simulink library "lib_fault_definiteness"  (R2023a)
settings: Solver=VariableStepAuto  StartTime=0.0  StopTime=10.0  RelTol=1e-3
settings Model: Creator=YXQ1WX  LastModifiedBy=xiaoqiang.yuan
settings OptimizationCC: ReuseModelBlockBuffer=off

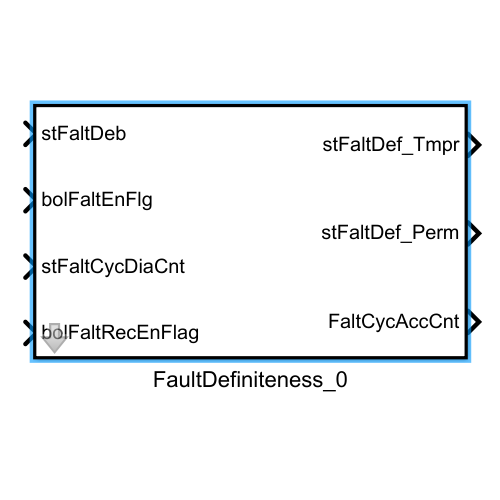
[thumbnail: Simulink's stored preview of the top-level diagram]
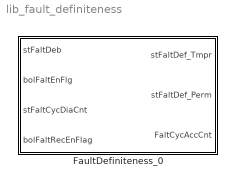
== system lib_fault_definiteness ==
  FaultDefiniteness_0 : Subsystem  TreatAsAtomicUnit=on  mask{lb_FaltWaitRecvCnt=0}
      mask prompts: lb_FaltWaitRecvCnt "FailWaitRecvryCounter"
      mask DialogControl DescGroupVar Prompt: WF control library
      mask DialogControl DescTextVar Prompt: For fault definiteness

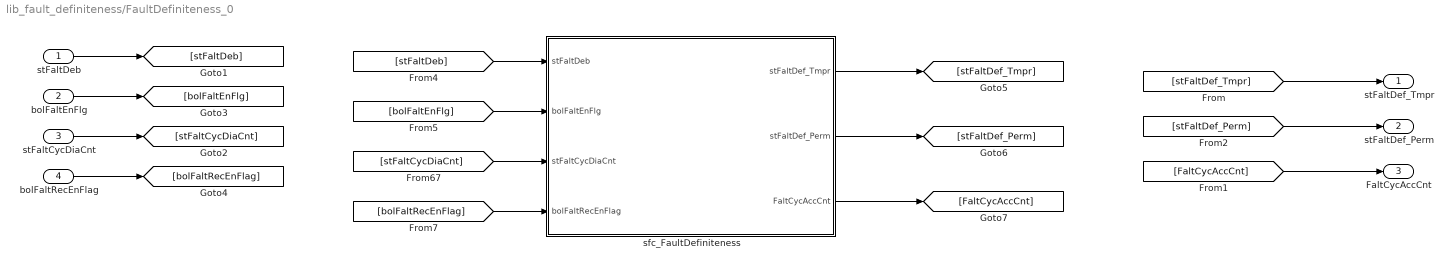
== system lib_fault_definiteness/FaultDefiniteness_0 ==
  stFaltDeb : Inport
  bolFaltEnFlg : Inport  Port=2
  stFaltCycDiaCnt : Inport  Port=3
  bolFaltRecEnFlag : Inport  Port=4
  sfc_FaultDefiniteness : Stateflow chart  TreatAsAtomicUnit=on
  stFaltDef_Tmpr : Outport
  stFaltDef_Perm : Outport  Port=2
  FaltCycAccCnt : Outport  Port=3
  wires:
  sfc_FaultDefiniteness/1(stFaltDef_Tmpr) -> [stFaltDef_Tmpr]
  sfc_FaultDefiniteness/2(stFaltDef_Perm) -> [stFaltDef_Perm]
  sfc_FaultDefiniteness/3(FaltCycAccCnt) -> [FaltCycAccCnt]
  [stFaltDeb] -> sfc_FaultDefiniteness/1(stFaltDeb)
  [bolFaltEnFlg] -> sfc_FaultDefiniteness/2(bolFaltEnFlg)
  [stFaltCycDiaCnt] -> sfc_FaultDefiniteness/3(stFaltCycDiaCnt)
  [bolFaltRecEnFlag] -> sfc_FaultDefiniteness/4(bolFaltRecEnFlag)
  stFaltDeb/1 -> [stFaltDeb]
  bolFaltEnFlg/1 -> [bolFaltEnFlg]
  stFaltCycDiaCnt/1 -> [stFaltCycDiaCnt]
  bolFaltRecEnFlag/1 -> [bolFaltRecEnFlag]
  [stFaltDef_Tmpr] -> stFaltDef_Tmpr/1
  [FaltCycAccCnt] -> FaltCycAccCnt/1
  [stFaltDef_Perm] -> stFaltDef_Perm/1

== stateflow chart lib_fault_definiteness/FaultDefiniteness_0/sfc_FaultDefiniteness ==
  state EnableDiagnosis
    state Normal
      /*Clear Bit0 Bit1*/
      en:  stFaltDef_Tmpr = false;
      stFaltDef_Perm = false;
      FaltCycAccCnt = uint8(0);
    state Confirming
      /*Set Bit0 Bit1*/
      en:  stFaltDef_Tmpr = true;
      stFaltDef_Perm = true;
      FaltCycAccCnt = FaltCycAccCnt + uint8(1);
    state Wait
      /*Set Bit0 Clear Bit1*/
      en:  stFaltDef_Tmpr = true;
      stFaltDef_Perm = false;
      FaltWaitRecvCnt = uint16(0);
      du:
      FaltWaitRecvCnt = FaltWaitRecvCnt + uint16(1);
      ex: FaltWaitRecvCnt = uint16(0);
    state Confirmed
      /*Set Bit1 Clear Bit0*/
      en:  stFaltDef_Tmpr = false;
      stFaltDef_Perm = true;
      FaltCycAccCnt = uint8(0);
    (default) -> Normal
    Normal -> (junction 181) : /*There is Fault*/
        | [stFaltDeb]
    (junction 181) -> (junction 184) [order 1] : /*Direct Confirm*/
        | [stFaltCycDiaCnt == uint8(0)]
    (junction 181) -> Confirming [order 2]
    (junction 184) -> Confirmed
    (junction 233) -> Normal
    Wait -> (junction 233) [order 2] : /*Confirm to Recovery*/
        | [FaltWaitRecvCnt > uint16(uint16(2*lb_FaltWaitRecvCnt) + uint16(100)) &&...
        | !stFaltDeb && bolFaltEnFlg]
    (junction 229) -> Normal
    Confirming -> Wait : /*There is no Fault*/
        | [!stFaltDeb]
    Wait -> (junction 212) [order 1] : /*There is Fault*/
        | [stFaltDeb]
    (junction 212) -> Confirming [order 2] : /*Need Confirm*/
    (junction 212) -> (junction 231) [order 1] : /*Fault is Confirmed*/
        | [FaltCycAccCnt >= stFaltCycDiaCnt]
    (junction 231) -> Confirmed
    Confirmed -> (junction 229) : /*Need Recovery*/
        | [bolFaltRecEnFlag &&...
        | !stFaltDeb]
  state DisableDiagnosis
    /*Clear Bit0 Bit1*/
    en:  stFaltDef_Tmpr = false;
    stFaltDef_Perm = false;
    FaltCycAccCnt = uint8(0);
  (default) -> DisableDiagnosis
  DisableDiagnosis -> EnableDiagnosis : /*Fault Need Enable*/
      | [bolFaltEnFlg]
  data: stFaltDeb input boolean; bolFaltEnFlg input boolean; stFaltCycDiaCnt input uint8; stFaltDef_Tmpr output boolean; bolFaltRecEnFlag input boolean; stFaltDef_Perm output boolean; FaltCycAccCnt output uint8; FaltWaitRecvCnt local uint16; lb_FaltWaitRecvCnt parameter
  data stFaltDeb settings: description=$TL$ inheritscaling=1; $TL$
  data bolFaltEnFlg settings: description=$TL$ inheritscaling=1; $TL$
  data stFaltCycDiaCnt settings: description=$TL$ inheritscaling=1; $TL$
  data stFaltDef_Tmpr settings: description=$TL$ type=UInt8; $TL$
  data bolFaltRecEnFlag settings: description=$TL$ inheritscaling=1; $TL$
  data stFaltDef_Perm settings: description=$TL$ type=UInt8; $TL$
  data FaltCycAccCnt settings: description=$TL$ type=UInt8; $TL$
  data FaltWaitRecvCnt settings: description=$TL$ type=UInt8; $TL$
  data lb_FaltWaitRecvCnt settings: description=$TL$ inheritscaling=1; $TL$
